simulink model "unicycle_control_template_R2018a_flocking"  (R2021b)
settings: Solver=ode45  StartTime=0.0  StopTime=15  RelTol=1e-5
PreLoadFcn:
  | % initialize variables
  | initializeUnicycleModel;
values from neighbouring files (symbols this model uses):
  c_ca = 1    [Project.m]
  c_fl = 5    [Project.m]
  c_g = 1    [Project.m]
  ic = [1,1,pi/2 ... (first row only)    [Project.m]
  R_ca = 3    [Project.m]
  Rn = 5    [Project.m]
  ugv_L = 2    [Project.m]
  v_max = 0.8*25    (= 20)    [Project.m]
  w_ca = 6    [Project.m]
  w_max = 3 * pi    (= 9.42477796077)    [Project.m]
settings Model: Creator=beniamino  LastModifiedBy=pool
settings SolverCC: ZeroCrossAlgorithm=Adaptive  AlgebraicLoopSolver=TrustRegion
settings DataIOCC: InitialState=cartesianInitialStates  SaveFormat=StructureWithTime  SaveOutput=off  SignalLogging=off  DSMLogging=off  SaveTime=off
settings DebuggingCC: IgnoredZcDiagnostic=none  ArithmeticOperatorsInVariantConditions=warning
settings SFSimCC: CustomCodeUndefinedFunction=UseInterfaceOnly

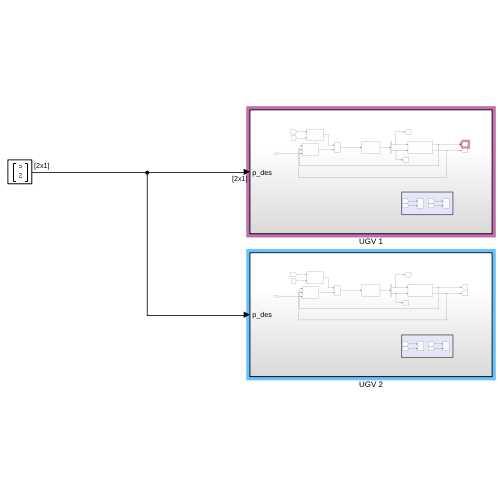
[thumbnail: Simulink's stored preview of the top-level diagram]
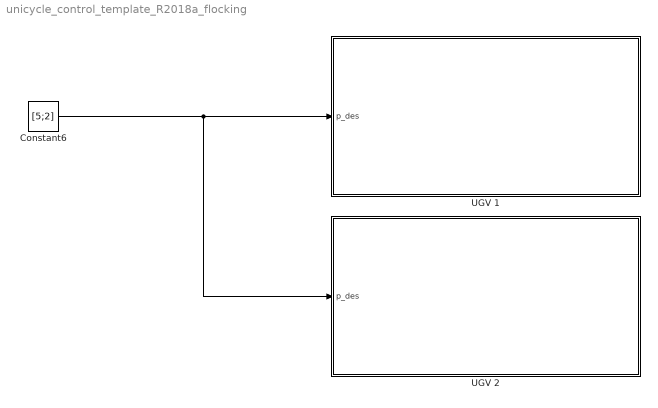
== system unicycle_control_template_R2018a_flocking ==
  Constant6 : Constant  Value=[5;2]  VectorParams1D=off
  UGV 1 : Subsystem
  UGV 2 : Subsystem
  wires:
  Constant6/1 -> UGV 2/1(p_des), UGV 1/1(p_des)

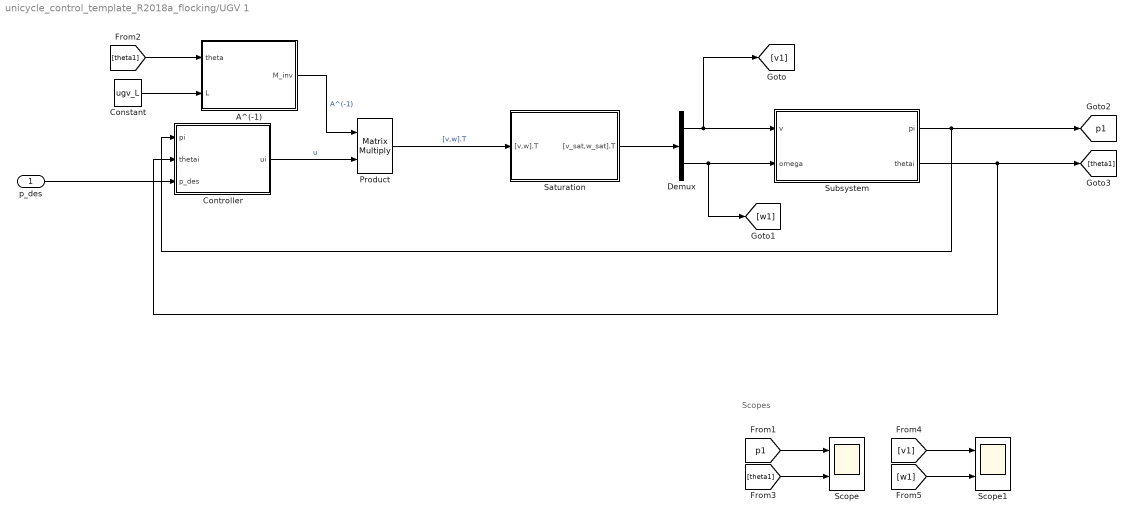
== system unicycle_control_template_R2018a_flocking/UGV 1 ==
  note: Scopes
  p_des : Inport
  A^(-1) : MATLAB Function  TreatAsAtomicUnit=on
  Constant : Constant  Value=ugv_L
  Controller : Subsystem
  Demux : Demux  Outputs=2
  Product : Product  Multiplication=Matrix(*)
  "Saturation " : Subsystem
  Scope : Scope  NumInputPorts=2
  Scope1 : Scope  NumInputPorts=2
  Subsystem : Subsystem
  tag scope: p1=global
  wires:
  "Saturation "/1("[v_sat,w_sat].T") -> Demux/1
  Product/1 -> "Saturation "/1("[v,w].T")  "[v,w].T"
  Demux/2 -> Subsystem/2(omega), [w1]
  [theta1] -> A^(-1)/1(theta)
  Demux/1 -> Subsystem/1(v), [v1]
  [v1] -> Scope1/1
  [theta1] -> Scope/2
  [w1] -> Scope1/2
  [p1] -> Scope/1
  Controller/1(ui) -> Product/2  "u"
  p_des/1 -> Controller/3(p_des)
  Constant/1 -> A^(-1)/2(L)
  A^(-1)/1(M_inv) -> Product/1  "A^(-1)"
  Subsystem/1(pi) -> Controller/1(pi), [p1]
  Subsystem/2(thetai) -> Controller/2(thetai), [theta1]

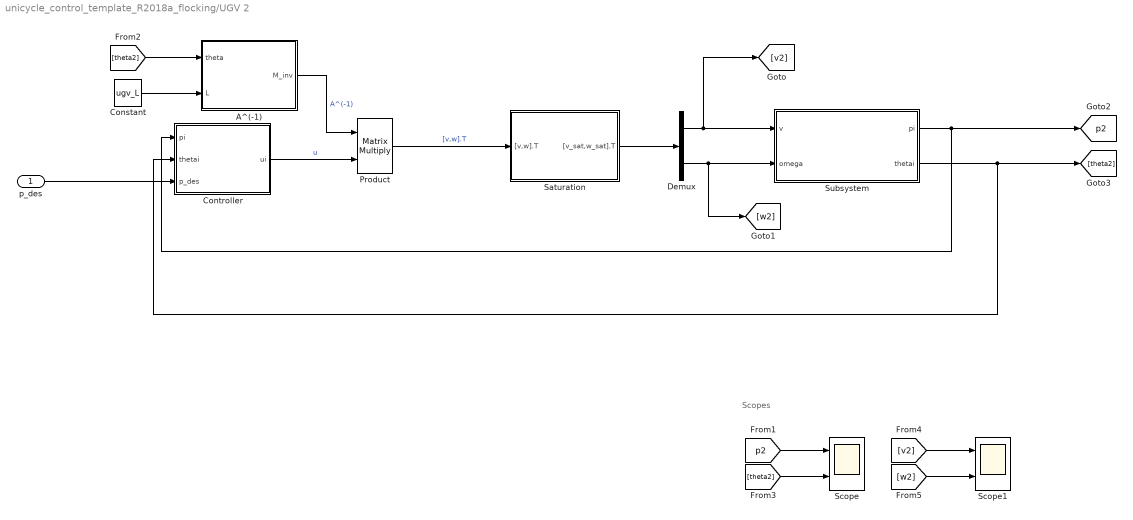
== system unicycle_control_template_R2018a_flocking/UGV 2 ==
  note: Scopes
  p_des : Inport
  A^(-1) : MATLAB Function  TreatAsAtomicUnit=on
  Constant : Constant  Value=ugv_L
  Controller : Subsystem
  Demux : Demux  Outputs=2
  Product : Product  Multiplication=Matrix(*)
  "Saturation " : Subsystem
  Scope : Scope  NumInputPorts=2
  Scope1 : Scope  NumInputPorts=2
  Subsystem : Subsystem
  tag scope: p2=global
  wires:
  "Saturation "/1("[v_sat,w_sat].T") -> Demux/1
  Product/1 -> "Saturation "/1("[v,w].T")  "[v,w].T"
  Demux/2 -> Subsystem/2(omega), [w2]
  [theta2] -> A^(-1)/1(theta)
  Demux/1 -> Subsystem/1(v), [v2]
  [v2] -> Scope1/1
  [theta2] -> Scope/2
  [w2] -> Scope1/2
  [p2] -> Scope/1
  Controller/1(ui) -> Product/2  "u"
  p_des/1 -> Controller/3(p_des)
  Constant/1 -> A^(-1)/2(L)
  A^(-1)/1(M_inv) -> Product/1  "A^(-1)"
  Subsystem/1(pi) -> Controller/1(pi), [p2]
  Subsystem/2(thetai) -> Controller/2(thetai), [theta2]

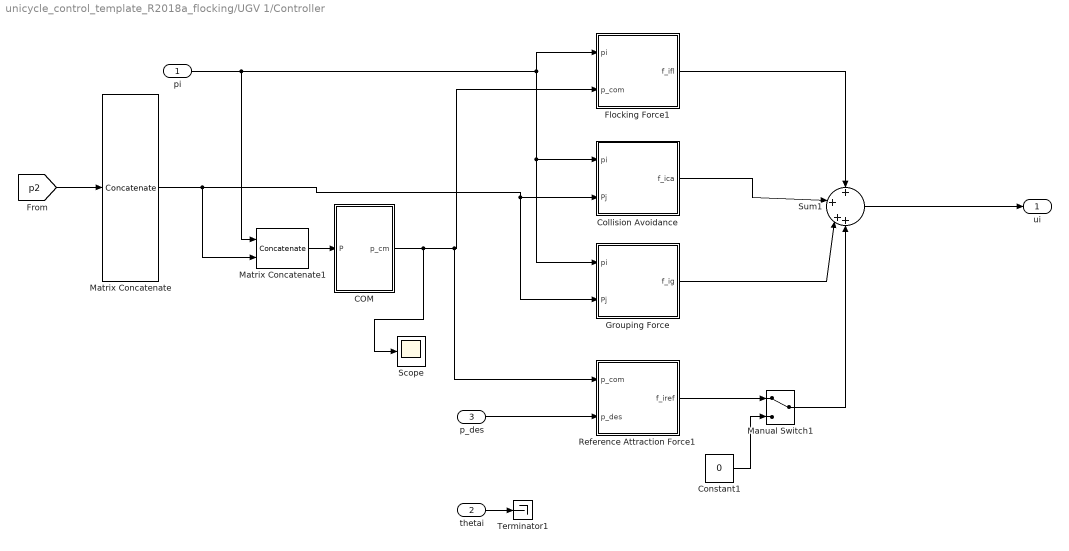
== system unicycle_control_template_R2018a_flocking/UGV 1/Controller ==
  pi : Inport
  thetai : Inport  Port=2
  p_des : Inport  Port=3
  COM : MATLAB Function  TreatAsAtomicUnit=on
  Collision Avoidance : Subsystem
  Constant1 : Constant  Value=0
  Flocking Force1 : Subsystem
  Grouping Force : Subsystem
  Manual Switch1 : ManualSwitch
  Matrix Concatenate : Concatenate  NumInputs=1  Mode=Multidimensional array  ConcatenateDimension=2
  Matrix Concatenate1 : Concatenate  Mode=Multidimensional array  ConcatenateDimension=2
  Reference Attraction Force1 : Subsystem
  Scope : Scope
  Sum1 : Sum  Inputs=+|+|++
  Terminator1 : Terminator
  ui : Outport
  wires:
  [p2] -> Matrix Concatenate/1
  COM/1(p_cm) -> Scope/1, Reference Attraction Force1/1(p_com), Flocking Force1/2(p_com)
  Grouping Force/1(f_ig) -> Sum1/3
  Manual Switch1/1 -> Sum1/4
  pi/1 -> Matrix Concatenate1/1, Grouping Force/1(pi), Collision Avoidance/1(pi), Flocking Force1/1(pi)
  thetai/1 -> Terminator1/1
  Constant1/1 -> Manual Switch1/2
  Collision Avoidance/1(f_ica) -> Sum1/2
  Flocking Force1/1(f_ifl) -> Sum1/1
  Reference Attraction Force1/1(f_iref) -> Manual Switch1/1
  Sum1/1 -> ui/1
  p_des/1 -> Reference Attraction Force1/2(p_des)
  Matrix Concatenate/1 -> Matrix Concatenate1/2, Grouping Force/2(Pj), Collision Avoidance/2(Pj)
  Matrix Concatenate1/1 -> COM/1(P)

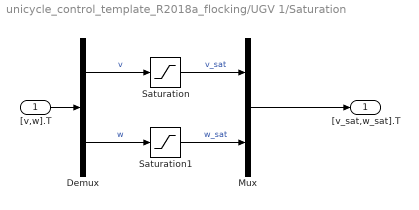
== system unicycle_control_template_R2018a_flocking/UGV 1/Saturation  ==
  "[v,w].T" : Inport
  Demux : Demux  Outputs=2
  Mux : Mux  Inputs=2
  Saturation : Saturate  UpperLimit=v_max  LowerLimit=0
  Saturation1 : Saturate  UpperLimit=w_max  LowerLimit=-w_max
  "[v_sat,w_sat].T" : Outport
  wires:
  "[v,w].T"/1 -> Demux/1
  Demux/1 -> Saturation/1  "v"
  Demux/2 -> Saturation1/1  "w"
  Saturation/1 -> Mux/1  "v_sat"
  Saturation1/1 -> Mux/2  "w_sat"
  Mux/1 -> "[v_sat,w_sat].T"/1

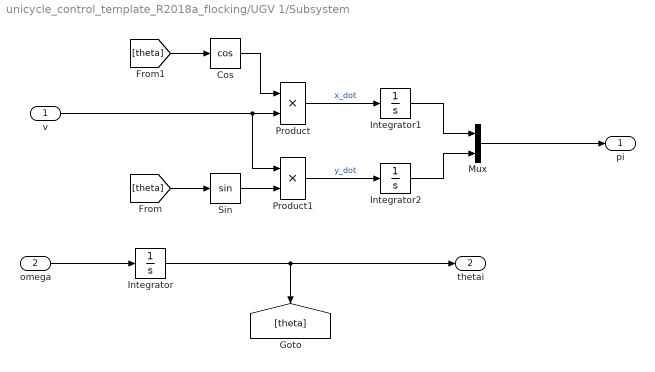
== system unicycle_control_template_R2018a_flocking/UGV 1/Subsystem ==
  v : Inport
  omega : Inport  Port=2
  Cos : Trigonometry  Operator=cos
  Integrator : Integrator  InitialCondition=ic(1,3)
  Integrator1 : Integrator  InitialCondition=ic(1,1)
  Integrator2 : Integrator  InitialCondition=ic(1,2)
  Mux : Mux  Inputs=2
  Product : Product
  Product1 : Product
  Sin : Trigonometry
  pi : Outport
  thetai : Outport  Port=2
  wires:
  Integrator/1 -> [theta], thetai/1
  Mux/1 -> pi/1
  v/1 -> Product1/1, Product/2
  omega/1 -> Integrator/1
  [theta] -> Sin/1
  [theta] -> Cos/1
  Cos/1 -> Product/1
  Sin/1 -> Product1/2
  Product/1 -> Integrator1/1  "x_dot"
  Product1/1 -> Integrator2/1  "y_dot"
  Integrator1/1 -> Mux/1
  Integrator2/1 -> Mux/2

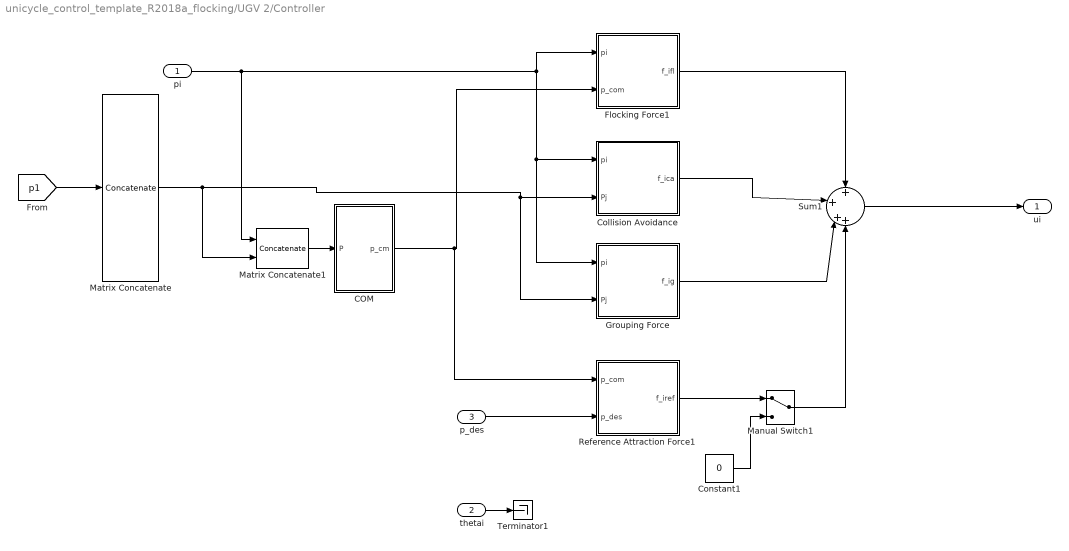
== system unicycle_control_template_R2018a_flocking/UGV 2/Controller ==
  pi : Inport
  thetai : Inport  Port=2
  p_des : Inport  Port=3
  COM : MATLAB Function  TreatAsAtomicUnit=on
  Collision Avoidance : Subsystem
  Constant1 : Constant  Value=0
  Flocking Force1 : Subsystem
  Grouping Force : Subsystem
  Manual Switch1 : ManualSwitch
  Matrix Concatenate : Concatenate  NumInputs=1  Mode=Multidimensional array  ConcatenateDimension=2
  Matrix Concatenate1 : Concatenate  Mode=Multidimensional array  ConcatenateDimension=2
  Reference Attraction Force1 : Subsystem
  Sum1 : Sum  Inputs=+|+|++
  Terminator1 : Terminator
  ui : Outport
  wires:
  [p1] -> Matrix Concatenate/1
  COM/1(p_cm) -> Reference Attraction Force1/1(p_com), Flocking Force1/2(p_com)
  Grouping Force/1(f_ig) -> Sum1/3
  Manual Switch1/1 -> Sum1/4
  pi/1 -> Matrix Concatenate1/1, Grouping Force/1(pi), Collision Avoidance/1(pi), Flocking Force1/1(pi)
  thetai/1 -> Terminator1/1
  Constant1/1 -> Manual Switch1/2
  Collision Avoidance/1(f_ica) -> Sum1/2
  Flocking Force1/1(f_ifl) -> Sum1/1
  Reference Attraction Force1/1(f_iref) -> Manual Switch1/1
  Sum1/1 -> ui/1
  p_des/1 -> Reference Attraction Force1/2(p_des)
  Matrix Concatenate/1 -> Matrix Concatenate1/2, Grouping Force/2(Pj), Collision Avoidance/2(Pj)
  Matrix Concatenate1/1 -> COM/1(P)

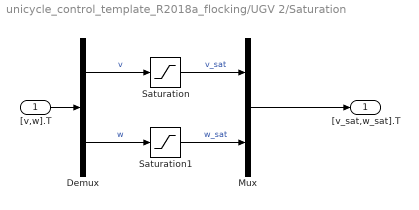
== system unicycle_control_template_R2018a_flocking/UGV 2/Saturation  ==
  "[v,w].T" : Inport
  Demux : Demux  Outputs=2
  Mux : Mux  Inputs=2
  Saturation : Saturate  UpperLimit=v_max  LowerLimit=0
  Saturation1 : Saturate  UpperLimit=w_max  LowerLimit=-w_max
  "[v_sat,w_sat].T" : Outport
  wires:
  "[v,w].T"/1 -> Demux/1
  Demux/1 -> Saturation/1  "v"
  Demux/2 -> Saturation1/1  "w"
  Saturation/1 -> Mux/1  "v_sat"
  Saturation1/1 -> Mux/2  "w_sat"
  Mux/1 -> "[v_sat,w_sat].T"/1

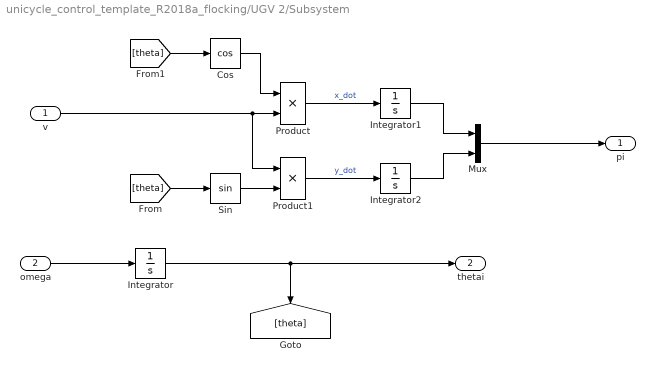
== system unicycle_control_template_R2018a_flocking/UGV 2/Subsystem ==
  v : Inport
  omega : Inport  Port=2
  Cos : Trigonometry  Operator=cos
  Integrator : Integrator  InitialCondition=ic(3,3)
  Integrator1 : Integrator  InitialCondition=ic(2,1)
  Integrator2 : Integrator  InitialCondition=ic(2,2)
  Mux : Mux  Inputs=2
  Product : Product
  Product1 : Product
  Sin : Trigonometry
  pi : Outport
  thetai : Outport  Port=2
  wires:
  Integrator/1 -> [theta], thetai/1
  Mux/1 -> pi/1
  v/1 -> Product1/1, Product/2
  omega/1 -> Integrator/1
  [theta] -> Sin/1
  [theta] -> Cos/1
  Cos/1 -> Product/1
  Sin/1 -> Product1/2
  Product/1 -> Integrator1/1  "x_dot"
  Product1/1 -> Integrator2/1  "y_dot"
  Integrator1/1 -> Mux/1
  Integrator2/1 -> Mux/2

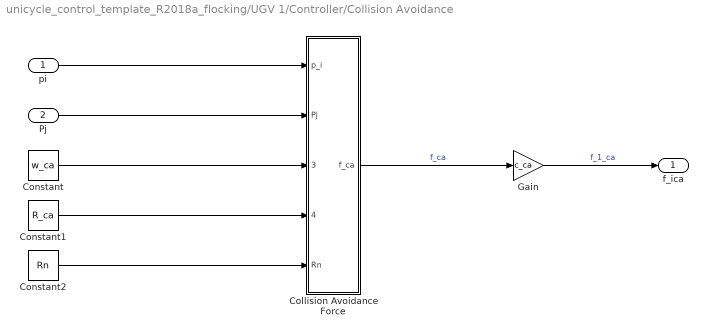
== system unicycle_control_template_R2018a_flocking/UGV 1/Controller/Collision Avoidance ==
  pi : Inport
  Pj : Inport  Port=2
  Collision Avoidance Force : MATLAB Function  TreatAsAtomicUnit=on
  Constant : Constant  Value=w_ca
  Constant1 : Constant  Value=R_ca
  Constant2 : Constant  Value=Rn
  Gain : Gain  Gain=c_ca
  f_ica : Outport
  wires:
  Collision Avoidance Force/1(f_ca) -> Gain/1  "f_ca"
  Gain/1 -> f_ica/1  "f_1_ca"
  Pj/1 -> Collision Avoidance Force/2(Pj)
  pi/1 -> Collision Avoidance Force/1(p_i)
  Constant/1 -> Collision Avoidance Force/3(w_ca)
  Constant1/1 -> Collision Avoidance Force/4(R_ca)
  Constant2/1 -> Collision Avoidance Force/5(Rn)

== system unicycle_control_template_R2018a_flocking/UGV 1/Controller/Flocking Force1 ==
  pi : Inport
  p_com : Inport  Port=2
  Gain : Gain  Gain=c_fl
  Sum : Sum  Inputs=-+
  f_ifl : Outport
  wires:
  pi/1 -> Sum/1
  p_com/1 -> Sum/2
  Sum/1 -> Gain/1  "pi_diff"
  Gain/1 -> f_ifl/1  "f_i_fl"

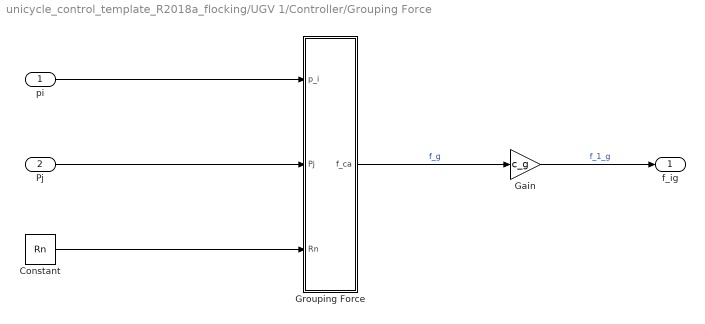
== system unicycle_control_template_R2018a_flocking/UGV 1/Controller/Grouping Force ==
  pi : Inport
  Pj : Inport  Port=2
  Constant : Constant  Value=Rn
  Gain : Gain  Gain=c_g
  Grouping Force : MATLAB Function  TreatAsAtomicUnit=on
  f_ig : Outport
  wires:
  Grouping Force/1(f_ca) -> Gain/1  "f_g"
  Gain/1 -> f_ig/1  "f_1_g"
  pi/1 -> Grouping Force/1(p_i)
  Pj/1 -> Grouping Force/2(Pj)
  Constant/1 -> Grouping Force/3(Rn)

== system unicycle_control_template_R2018a_flocking/UGV 1/Controller/Reference Attraction Force1 ==
  p_com : Inport
  p_des : Inport  Port=2
  Gain : Gain  Gain=10
  Sum : Sum  Inputs=-+
  f_iref : Outport
  wires:
  Sum/1 -> Gain/1  "f_ref"
  Gain/1 -> f_iref/1  "f_1_ref"
  p_des/1 -> Sum/2
  p_com/1 -> Sum/1

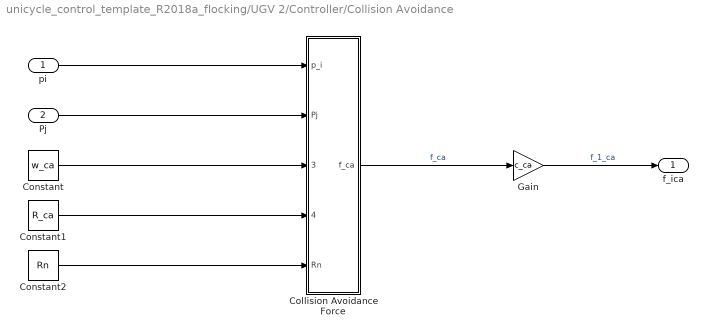
== system unicycle_control_template_R2018a_flocking/UGV 2/Controller/Collision Avoidance ==
  pi : Inport
  Pj : Inport  Port=2
  Collision Avoidance Force : MATLAB Function  TreatAsAtomicUnit=on
  Constant : Constant  Value=w_ca
  Constant1 : Constant  Value=R_ca
  Constant2 : Constant  Value=Rn
  Gain : Gain  Gain=c_ca
  f_ica : Outport
  wires:
  Collision Avoidance Force/1(f_ca) -> Gain/1  "f_ca"
  Gain/1 -> f_ica/1  "f_1_ca"
  Pj/1 -> Collision Avoidance Force/2(Pj)
  pi/1 -> Collision Avoidance Force/1(p_i)
  Constant/1 -> Collision Avoidance Force/3(w_ca)
  Constant1/1 -> Collision Avoidance Force/4(R_ca)
  Constant2/1 -> Collision Avoidance Force/5(Rn)

== system unicycle_control_template_R2018a_flocking/UGV 2/Controller/Flocking Force1 ==
  pi : Inport
  p_com : Inport  Port=2
  Gain : Gain  Gain=c_fl
  Sum : Sum  Inputs=-+
  f_ifl : Outport
  wires:
  pi/1 -> Sum/1
  p_com/1 -> Sum/2
  Sum/1 -> Gain/1  "pi_diff"
  Gain/1 -> f_ifl/1  "f_i_fl"

== system unicycle_control_template_R2018a_flocking/UGV 2/Controller/Grouping Force ==
  pi : Inport
  Pj : Inport  Port=2
  Constant : Constant  Value=Rn
  Gain : Gain  Gain=c_g
  Grouping Force : MATLAB Function  TreatAsAtomicUnit=on
  f_ig : Outport
  wires:
  Grouping Force/1(f_ca) -> Gain/1  "f_g"
  Gain/1 -> f_ig/1  "f_1_g"
  pi/1 -> Grouping Force/1(p_i)
  Pj/1 -> Grouping Force/2(Pj)
  Constant/1 -> Grouping Force/3(Rn)

== system unicycle_control_template_R2018a_flocking/UGV 2/Controller/Reference Attraction Force1 ==
  p_com : Inport
  p_des : Inport  Port=2
  Gain : Gain  Gain=10
  Sum : Sum  Inputs=-+
  f_iref : Outport
  wires:
  Sum/1 -> Gain/1  "f_ref"
  Gain/1 -> f_iref/1  "f_1_ref"
  p_des/1 -> Sum/2
  p_com/1 -> Sum/1

== matlab function unicycle_control_template_R2018a_flocking/UGV 2/A^(-1) ==
  data: theta input; M_inv output; L input
function M_inv = A_inv(theta, L)
    % This function returns the inverse "state matrix" evaluated at the current
    % theta
    M = [cos(theta), -L * sin(theta); 
        sin(theta), L*cos(theta)];
    % Notice that M is always invertible
M_inv = M^(-1);

== matlab function unicycle_control_template_R2018a_flocking/UGV 2/Controller/COM ==
  data: P input; p_cm output
function p_cm = fcn(P)
p_cm = mean(P,2);

== matlab function unicycle_control_template_R2018a_flocking/UGV 2/Controller/Collision Avoidance/Collision Avoidance Force ==
  data: p_i input; f_ca output; Pj input; w_ca input; R_ca input; Rn input
function f_ca = fcn(p_i,Pj, w_ca, R_ca, Rn)

% Create the contribution for the detected UGV's (closer than R_n)
total = zeros(2,1);
dims = size(Pj);

columns = dims(2);
for i=1:columns
    pj = Pj(:,i);
    if(norm(p_i-pj) <= Rn)                                       % We have detected another UGV nearby
        direction = (p_i - pj) / norm(p_i -pj);                   % Direction toward we need to move
        weight = 1/(1 + exp(w_ca * (norm(p_i-pj) - R_ca)));      % Weight more the closer we are to another UGV
        total = total + weight * direction; 
    end
end

f_ca = total;

== matlab function unicycle_control_template_R2018a_flocking/UGV 2/Controller/Grouping Force/Grouping Force ==
  data: p_i input; f_ca output; Pj input; Rn input
function f_ca = fcn(p_i,Pj, Rn)

% Create the contribution for the detected UGV's (closer than R_n)
total = zeros(2,1);
dims = size(Pj);
columns = dims(2);
for i=1:columns
    pj = Pj(:,i);
    if(norm(p_i-pj) <= Rn)          % We have detected another UGV nearby
        total = total + (pj - p_i);
    end
end
f_ca = total;

== matlab function unicycle_control_template_R2018a_flocking/UGV 1/A^(-1) ==
  data: theta input; M_inv output; L input
function M_inv = A_inv(theta, L)
    % This function returns the inverse "state matrix" evaluated at the current
    % theta
    M = [cos(theta), -L * sin(theta); 
        sin(theta), L*cos(theta)];
    % Notice that M is always invertible
M_inv = M^(-1);

== matlab function unicycle_control_template_R2018a_flocking/UGV 1/Controller/COM ==
  data: P input; p_cm output
function p_cm = fcn(P)
p_cm = mean(P,2);

== matlab function unicycle_control_template_R2018a_flocking/UGV 1/Controller/Collision Avoidance/Collision Avoidance Force ==
  data: p_i input; f_ca output; Pj input; w_ca input; R_ca input; Rn input
function f_ca = fcn(p_i,Pj, w_ca, R_ca, Rn)

% Create the contribution for the detected UGV's (closer than R_n)
total = zeros(2,1);
dims = size(Pj);

columns = dims(2);
for i=1:columns
    pj = Pj(:,i);
    if(norm(p_i-pj) <= Rn)                                       % We have detected another UGV nearby
        direction = (p_i - pj) / norm(p_i -pj);                   % Direction toward we need to move
        weight = 1/(1 + exp(w_ca * (norm(p_i-pj) - R_ca)));      % Weight more the closer we are to another UGV
        total = total + weight * direction; 
    end
end

f_ca = total;

== matlab function unicycle_control_template_R2018a_flocking/UGV 1/Controller/Grouping Force/Grouping Force ==
  data: p_i input; f_ca output; Pj input; Rn input
function f_ca = fcn(p_i,Pj, Rn)

% Create the contribution for the detected UGV's (closer than R_n)
total = zeros(2,1);
dims = size(Pj);
columns = dims(2);
for i=1:columns
    pj = Pj(:,i);
    if(norm(p_i-pj) <= Rn)          % We have detected another UGV nearby
        total = total + (pj - p_i);
    end
end
f_ca = total;
